simulink model "ModelCurrentState"  (R2024b)
settings: Solver=VariableStepAuto  StartTime=0.0  StopTime=StopTime  MaxStep=0.001  RelTol=1e-3
model workspace: external: MAT-File 3DModelInputs.mat (data not in the file)
undefined symbols (not defined in the file): GripStrength, KillswitchFinalValue, KillswitchInitialValue, KillswitchStepTime, LeftLowerArmLength, PlaneTilt, RightLowerArmLength, UpperTorsoLength, X, Y, Z
libraries: nesl_utility x408, sm_lib x139, matrix_library x11, simulink x1
(part 5 of 14)

== system ModelCurrentState/Right Shoulder Joint ==
  note: RSGlobal
  Dot Product1 : DotProduct  OutDataTypeStr=Inherit: Inherit via internal rule
  Dot Product2 : DotProduct  OutDataTypeStr=Inherit: Inherit via internal rule
  RArmonRSFGlobal : Gain  Gain=-1
  RArmonRSTGlobal : Gain  Gain=-1
  RS Kinematically Driven : Subsystem  Commented=on
  RS Kinetically Driven : Subsystem
  RSAV : nesl_utility/PS-Simulink Converter  PhysicalDomain=network_engine_domain  SubClassName=ps_output  LeftPortType=input  RightPortType=output  PseudoPeriodic=off  Frequencies=[]  VectorFormat=1-D array  Unit=deg/s  AffineConversion=off
  RSAngularWorkonArm : Integrator
  RSLinearImpulseonArm : Integrator
  RSLinearWorkonArm : Integrator
  RSgx : nesl_utility/PS-Simulink Converter  PhysicalDomain=network_engine_domain  SubClassName=ps_output  LeftPortType=input  RightPortType=output  PseudoPeriodic=off  Frequencies=[]  VectorFormat=1-D array  Unit=inherit  AffineConversion=off
  RSgy : nesl_utility/PS-Simulink Converter  PhysicalDomain=network_engine_domain  SubClassName=ps_output  LeftPortType=input  RightPortType=output  PseudoPeriodic=off  Frequencies=[]  VectorFormat=1-D array  Unit=inherit  AffineConversion=off
  RSgz : nesl_utility/PS-Simulink Converter  PhysicalDomain=network_engine_domain  SubClassName=ps_output  LeftPortType=input  RightPortType=output  PseudoPeriodic=off  Frequencies=[]  VectorFormat=1-D array  Unit=inherit  AffineConversion=off
  RSonRArmFGlob : Product  Multiplication=Matrix(*)
  RSonRArmLocalForce : nesl_utility/PS-Simulink Converter  PhysicalDomain=network_engine_domain  SubClassName=ps_output  LeftPortType=input  RightPortType=output  PseudoPeriodic=off  Frequencies=[]  VectorFormat=1-D array  Unit=inherit  AffineConversion=off
  RSonRArmLocalTorque : nesl_utility/PS-Simulink Converter  PhysicalDomain=network_engine_domain  SubClassName=ps_output  LeftPortType=input  RightPortType=output  PseudoPeriodic=off  Frequencies=[]  VectorFormat=1-D array  Unit=inherit  AffineConversion=off
  RSonRArmTGlobal : Product  Multiplication=Matrix(*)
  RSvGlobal : nesl_utility/PS-Simulink Converter  PhysicalDomain=network_engine_domain  SubClassName=ps_output  LeftPortType=input  RightPortType=output  PseudoPeriodic=off  Frequencies=[]  VectorFormat=1-D array  Unit=inherit  AffineConversion=off
  RSx : nesl_utility/PS-Simulink Converter  PhysicalDomain=network_engine_domain  SubClassName=ps_output  LeftPortType=input  RightPortType=output  PseudoPeriodic=off  Frequencies=[]  VectorFormat=1-D array  Unit=inherit  AffineConversion=off
  RSy : nesl_utility/PS-Simulink Converter  PhysicalDomain=network_engine_domain  SubClassName=ps_output  LeftPortType=input  RightPortType=output  PseudoPeriodic=off  Frequencies=[]  VectorFormat=1-D array  Unit=inherit  AffineConversion=off
  RSz : nesl_utility/PS-Simulink Converter  PhysicalDomain=network_engine_domain  SubClassName=ps_output  LeftPortType=input  RightPortType=output  PseudoPeriodic=off  Frequencies=[]  VectorFormat=1-D array  Unit=inherit  AffineConversion=off
  RotationMatrix : nesl_utility/PS-Simulink Converter  PhysicalDomain=network_engine_domain  SubClassName=ps_output  LeftPortType=input  RightPortType=output  PseudoPeriodic=off  Frequencies=[]  VectorFormat=1-D array  Unit=inherit  AffineConversion=off
  Spherical Solid : sm_lib/Body Elements/Spherical Solid  SphereRadius=1.75  SphereRadiusUnits=in  ExportEntireGeometry=off  InertiaType=CalculateFromGeometry  BasedOnType=Density  Density=0  DensityUnits=kg/m^3  Mass=1  MassUnits=kg  CenterOfMass=[0 0 0]  CenterOfMassUnits=m  MomentsOfInertia=[1 1 1]  MomentsOfInertiaUnits=kg*m^2  ProductsOfInertia=[0 0 0]  ProductsOfInertiaUnits=kg*m^2  GraphicType=FromGeometry  MarkerShape=Sphere  MarkerSize=10  GraphicVisPropType=SimpleVisualProperties  GraphicDiffuseColor=[0.2 0.2 1.0]  GraphicOpacity=1  GraphicSpecularColor=[0.5 0.5 0.5 1.0]  GraphicAmbientColor=[0.15 0.15 0.15 1.0]  GraphicEmissiveColor=[0.0 0.0 0.0 1.0]  GraphicShininess=75  DoExposeReferenceFrame=on  SerializedFrames=<Frames/>
  Transform Sensor : sm_lib/Frames and Transforms/Transform Sensor  MeasurementFrame=World  RotationSequence=XYX  SenseAngle=off  SenseAxis=off  SenseQ=off  SenseR=on  SenseRotationSequence=off  SenseOmegaX=off  SenseOmegaY=off  SenseOmegaZ=off  SenseOmega=off  SenseQDot=off  SenseRDot=off  SenseRotationSequenceDot=off  SenseAlphaX=off  SenseAlphaY=off  SenseAlphaZ=off  SenseAlpha=off  SenseQDDot=off  SenseRDDot=off  SenseX=on  SenseY=on  SenseZ=on  SenseXYZ=off  SenseRad=off  SenseAzim=off  SenseDist=off  SenseInc=off  SenseXDot=off  SenseYDot=off  SenseZDot=off  SenseXYZDot=off  SenseRadDot=off  SenseAzimDot=off  SenseDistDot=off  SenseIncDot=off  SenseXDDot=off  SenseYDDot=off  SenseZDDot=off  SenseXYZDDot=off  SenseRadDDot=off  SenseAzimDDot=off  SenseDistDDot=off  SenseIncDDot=off
  Transform Sensor1 : sm_lib/Frames and Transforms/Transform Sensor  MeasurementFrame=World  RotationSequence=XYX  SenseAngle=off  SenseAxis=off  SenseQ=off  SenseR=off  SenseRotationSequence=off  SenseOmegaX=off  SenseOmegaY=off  SenseOmegaZ=off  SenseOmega=on  SenseQDot=off  SenseRDot=off  SenseRotationSequenceDot=off  SenseAlphaX=off  SenseAlphaY=off  SenseAlphaZ=off  SenseAlpha=off  SenseQDDot=off  SenseRDDot=off  SenseX=on  SenseY=on  SenseZ=on  SenseXYZ=off  SenseRad=off  SenseAzim=off  SenseDist=off  SenseInc=off  SenseXDot=off  SenseYDot=off  SenseZDot=off  SenseXYZDot=on  SenseRadDot=off  SenseAzimDot=off  SenseDistDot=off  SenseIncDot=off  SenseXDDot=off  SenseYDDot=off  SenseZDDot=off  SenseXYZDDot=off  SenseRadDDot=off  SenseAzimDDot=off  SenseDistDDot=off  SenseIncDDot=off
  Vector Concatenate : Concatenate  NumInputs=3
  World Frame : sm_lib/Frames and Transforms/World Frame
  Right Shoulder : PMIOPort  Side=Left
  Top of Right Arm : PMIOPort  Port=2  Side=Right
  tag scope: RSGlobalPosition=global, RSonRArmFGlobalOut=global, RSonRArmTGlobalOut=global
  wires:
  RotationMatrix/1 -> RSonRArmFGlob/1, RSonRArmTGlobal/1
  RSonRArmLocalForce/1 -> RSonRArmFGlob/2
  RSonRArmLocalTorque/1 -> RSonRArmTGlobal/2
  RSonRArmTGlobal/1 -> Dot Product2/1, RArmonRSTGlobal/1, [RSonRArmTGlobalOut]  "RSonRArmTGlobal"
  RSgx/1 -> Vector Concatenate/1
  RSgy/1 -> Vector Concatenate/2
  Vector Concatenate/1 -> [RSGlobalPosition]  "RSGlobalPosition"
  RSgz/1 -> Vector Concatenate/3
  Dot Product1/1 -> RSLinearWorkonArm/1  "RSonArmLinearPower"
  Dot Product2/1 -> RSAngularWorkonArm/1  "RSonArmAngularPower"
  RSonRArmFGlob/1 -> RSLinearImpulseonArm/1, Dot Product1/1, [RSonRArmFGlobalOut], RArmonRSFGlobal/1  "RSonRArmFGlobal"
  RSvGlobal/1 -> Dot Product1/2  "RSVGlobal"
  RSAV/1 -> Dot Product2/2  "RSAVGlobal"
  connections:
  Spherical Solid/RConn1 -- RS Kinetically Driven/LConn1 -- Top of Right Arm/RConn1 -- RS Kinematically Driven/LConn1 -- Transform Sensor1/RConn1 -- Transform Sensor/RConn1
  RSgx/LConn1 -- Transform Sensor/RConn3
  RotationMatrix/LConn1 -- Transform Sensor/RConn2
  RSgz/LConn1 -- Transform Sensor/RConn5
  RSgy/LConn1 -- Transform Sensor/RConn4
  World Frame/RConn1 -- Transform Sensor1/LConn1 -- Transform Sensor/LConn1
  Transform Sensor1/RConn6 -- RSvGlobal/LConn1
  RSAV/LConn1 -- Transform Sensor1/RConn2
  Transform Sensor1/RConn5 -- RSz/LConn1
  Transform Sensor1/RConn4 -- RSy/LConn1
  Transform Sensor1/RConn3 -- RSx/LConn1
  RS Kinematically Driven/RConn1 -- Right Shoulder/RConn1 -- RS Kinetically Driven/RConn1
  RSonRArmLocalForce/LConn1 -- RS Kinetically Driven/RConn2
  RSonRArmLocalTorque/LConn1 -- RS Kinetically Driven/RConn3

== system ModelCurrentState/Right Upper Arm ==
  Cylindrical Solid3 : sm_lib/Body Elements/Cylindrical Solid  CylinderRadius=1.75  CylinderRadiusUnits=in  CylinderLength=12  CylinderLengthUnits=in  ExportEntireGeometry=off  InertiaType=CalculateFromGeometry  BasedOnType=Mass  Density=1000  DensityUnits=kg/m^3  Mass=5  MassUnits=lbm  CenterOfMass=[0 0 0]  CenterOfMassUnits=m  MomentsOfInertia=[1 1 1]  MomentsOfInertiaUnits=kg*m^2  ProductsOfInertia=[0 0 0]  ProductsOfInertiaUnits=kg*m^2  GraphicType=FromGeometry  MarkerShape=Sphere  MarkerSize=10  GraphicVisPropType=SimpleVisualProperties  GraphicDiffuseColor=[0.2 0.2 1.0]  GraphicOpacity=1.0  GraphicSpecularColor=[0.5 0.5 0.5 1.0]  GraphicAmbientColor=[0.15 0.15 0.15 1.0]  GraphicEmissiveColor=[0.0 0.0 0.0 1.0]  GraphicShininess=75  DoExposeReferenceFrame=off  SerializedFrames=<Frames><Frame><Id>Frame1</Id><Value><Name>Top of Right Arm</Name><Origin><Source>GeometricFeature</Source><FeatureName>top curve</FeatureName></Origin><PrimaryAxis><DefinedDirection>-X</DefinedDirection><Source>ReferenceFrame</Source><SourceDirection>+Z</SourceDirection><FeatureName></FeatureName></PrimaryAxis><SecondaryAxis><DefinedDirection>+Y</DefinedDirection><Source>ReferenceFrame</Source><SourceDirection>+X</SourceDirection><FeatureName></FeatureName></SecondaryAxis></Value></Frame><Frame><Id>Frame2</Id><Value><Name>Bottom of Right Arm</Name><Origin><Source>GeometricFeature</Source><FeatureName>bottom curve</FeatureName></Origin><PrimaryAxis><DefinedDirection>-X</DefinedDirection><Source>ReferenceFrame</Source><SourceDirection>+Z</SourceDirection><FeatureName></FeatureName></PrimaryAxis><SecondaryAxis><DefinedDirection>+Z</DefinedDirection><Source>ReferenceFrame</Source><SourceDirection>-X</SourceDirection><FeatureName></FeatureName></SecondaryAxis></Value></Frame></Frames>
  Right Upper Arm MOF : Subsystem  Commented=on
  RightUpper  Arm : PMIOPort  Side=Left
  Right Elbow : PMIOPort  Port=2  Side=Right
  connections:
  Right Upper Arm MOF/LConn1 -- RightUpper  Arm/RConn1 -- Cylindrical Solid3/LConn1
  Cylindrical Solid3/RConn1 -- Right Elbow/RConn1

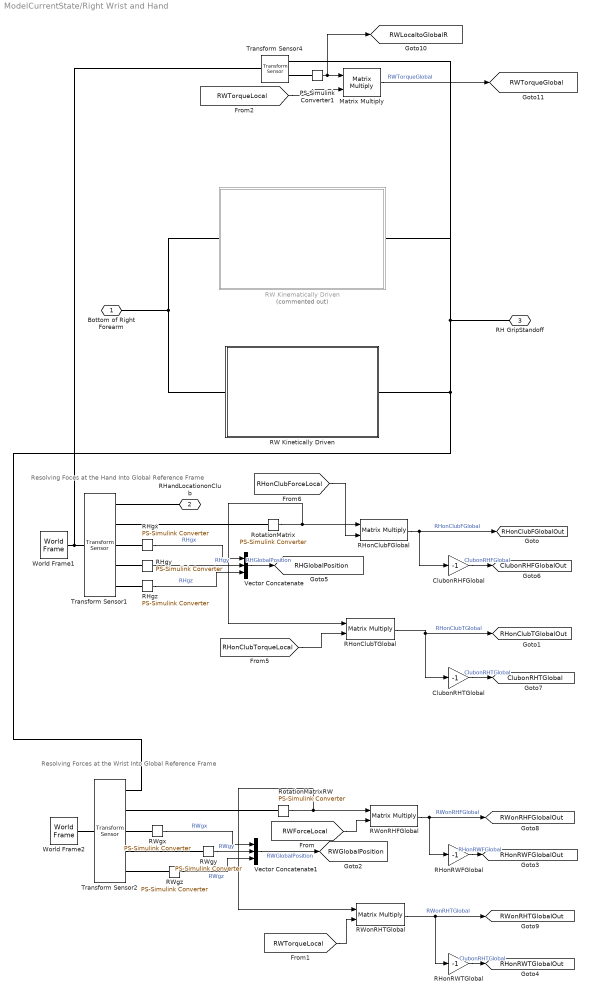
== system ModelCurrentState/Right Wrist and Hand ==
  note: Resolving Foces at the Hand Into Global Reference Frame
  note: Resolving Forces at the Wrist Into Global Reference Frame
  ClubonRHFGlobal : Gain  Gain=-1
  ClubonRHTGlobal : Gain  Gain=-1
  Matrix Multiply : Product  Multiplication=Matrix(*)
  PS-Simulink Converter1 : nesl_utility/PS-Simulink Converter  PhysicalDomain=network_engine_domain  SubClassName=ps_output  LeftPortType=input  RightPortType=output  PseudoPeriodic=off  Frequencies=[]  VectorFormat=1-D array  Unit=inherit  AffineConversion=off
  RHgx : nesl_utility/PS-Simulink Converter  PhysicalDomain=network_engine_domain  SubClassName=ps_output  LeftPortType=input  RightPortType=output  PseudoPeriodic=off  Frequencies=[]  VectorFormat=1-D array  Unit=inherit  AffineConversion=off
  RHgy : nesl_utility/PS-Simulink Converter  PhysicalDomain=network_engine_domain  SubClassName=ps_output  LeftPortType=input  RightPortType=output  PseudoPeriodic=off  Frequencies=[]  VectorFormat=1-D array  Unit=inherit  AffineConversion=off
  RHgz : nesl_utility/PS-Simulink Converter  PhysicalDomain=network_engine_domain  SubClassName=ps_output  LeftPortType=input  RightPortType=output  PseudoPeriodic=off  Frequencies=[]  VectorFormat=1-D array  Unit=inherit  AffineConversion=off
  RHonClubFGlobal : Product  Multiplication=Matrix(*)
  RHonClubTGlobal : Product  Multiplication=Matrix(*)
  RHonRWFGlobal : Gain  Gain=-1
  RHonRWTGlobal : Gain  Gain=-1
  RW Kinematically Driven : Subsystem  Commented=on
  RW Kinetically Driven : Subsystem
  RWgx : nesl_utility/PS-Simulink Converter  PhysicalDomain=network_engine_domain  SubClassName=ps_output  LeftPortType=input  RightPortType=output  PseudoPeriodic=off  Frequencies=[]  VectorFormat=1-D array  Unit=inherit  AffineConversion=off
  RWgy : nesl_utility/PS-Simulink Converter  PhysicalDomain=network_engine_domain  SubClassName=ps_output  LeftPortType=input  RightPortType=output  PseudoPeriodic=off  Frequencies=[]  VectorFormat=1-D array  Unit=inherit  AffineConversion=off
  RWgz : nesl_utility/PS-Simulink Converter  PhysicalDomain=network_engine_domain  SubClassName=ps_output  LeftPortType=input  RightPortType=output  PseudoPeriodic=off  Frequencies=[]  VectorFormat=1-D array  Unit=inherit  AffineConversion=off
  RWonRHFGlobal : Product  Multiplication=Matrix(*)
  RWonRHTGlobal : Product  Multiplication=Matrix(*)
  RotationMatrix : nesl_utility/PS-Simulink Converter  PhysicalDomain=network_engine_domain  SubClassName=ps_output  LeftPortType=input  RightPortType=output  PseudoPeriodic=off  Frequencies=[]  VectorFormat=1-D array  Unit=inherit  AffineConversion=off
  RotationMatrixRW : nesl_utility/PS-Simulink Converter  PhysicalDomain=network_engine_domain  SubClassName=ps_output  LeftPortType=input  RightPortType=output  PseudoPeriodic=off  Frequencies=[]  VectorFormat=1-D array  Unit=inherit  AffineConversion=off
  Transform Sensor1 : sm_lib/Frames and Transforms/Transform Sensor  MeasurementFrame=World  RotationSequence=XYX  SenseAngle=off  SenseAxis=off  SenseQ=off  SenseR=on  SenseRotationSequence=off  SenseOmegaX=off  SenseOmegaY=off  SenseOmegaZ=off  SenseOmega=off  SenseQDot=off  SenseRDot=off  SenseRotationSequenceDot=off  SenseAlphaX=off  SenseAlphaY=off  SenseAlphaZ=off  SenseAlpha=off  SenseQDDot=off  SenseRDDot=off  SenseX=on  SenseY=on  SenseZ=on  SenseXYZ=off  SenseRad=off  SenseAzim=off  SenseDist=off  SenseInc=off  SenseXDot=off  SenseYDot=off  SenseZDot=off  SenseXYZDot=off  SenseRadDot=off  SenseAzimDot=off  SenseDistDot=off  SenseIncDot=off  SenseXDDot=off  SenseYDDot=off  SenseZDDot=off  SenseXYZDDot=off  SenseRadDDot=off  SenseAzimDDot=off  SenseDistDDot=off  SenseIncDDot=off
  Transform Sensor2 : sm_lib/Frames and Transforms/Transform Sensor  MeasurementFrame=World  RotationSequence=XYX  SenseAngle=off  SenseAxis=off  SenseQ=off  SenseR=on  SenseRotationSequence=off  SenseOmegaX=off  SenseOmegaY=off  SenseOmegaZ=off  SenseOmega=off  SenseQDot=off  SenseRDot=off  SenseRotationSequenceDot=off  SenseAlphaX=off  SenseAlphaY=off  SenseAlphaZ=off  SenseAlpha=off  SenseQDDot=off  SenseRDDot=off  SenseX=on  SenseY=on  SenseZ=on  SenseXYZ=off  SenseRad=off  SenseAzim=off  SenseDist=off  SenseInc=off  SenseXDot=off  SenseYDot=off  SenseZDot=off  SenseXYZDot=off  SenseRadDot=off  SenseAzimDot=off  SenseDistDot=off  SenseIncDot=off  SenseXDDot=off  SenseYDDot=off  SenseZDDot=off  SenseXYZDDot=off  SenseRadDDot=off  SenseAzimDDot=off  SenseDistDDot=off  SenseIncDDot=off
  Transform Sensor4 : sm_lib/Frames and Transforms/Transform Sensor  MeasurementFrame=World  RotationSequence=XYX  SenseAngle=off  SenseAxis=off  SenseQ=off  SenseR=on  SenseRotationSequence=off  SenseOmegaX=off  SenseOmegaY=off  SenseOmegaZ=off  SenseOmega=off  SenseQDot=off  SenseRDot=off  SenseRotationSequenceDot=off  SenseAlphaX=off  SenseAlphaY=off  SenseAlphaZ=off  SenseAlpha=off  SenseQDDot=off  SenseRDDot=off  SenseX=off  SenseY=off  SenseZ=off  SenseXYZ=off  SenseRad=off  SenseAzim=off  SenseDist=off  SenseInc=off  SenseXDot=off  SenseYDot=off  SenseZDot=off  SenseXYZDot=off  SenseRadDot=off  SenseAzimDot=off  SenseDistDot=off  SenseIncDot=off  SenseXDDot=off  SenseYDDot=off  SenseZDDot=off  SenseXYZDDot=off  SenseRadDDot=off  SenseAzimDDot=off  SenseDistDDot=off  SenseIncDDot=off
  Vector Concatenate : Concatenate  NumInputs=3
  Vector Concatenate1 : Concatenate  NumInputs=3
  World Frame1 : sm_lib/Frames and Transforms/World Frame
  World Frame2 : sm_lib/Frames and Transforms/World Frame
  Bottom of Right Forearm : PMIOPort  Side=Left
  RHandLocationonClub : PMIOPort  Port=2  Side=Right
  RH GripStandoff : PMIOPort  Port=3  Side=Right
  tag scope: ClubonRHFGlobalOut=global, ClubonRHTGlobal=global, RHGlobalPosition=global, RHonClubFGlobalOut=global, RHonClubTGlobalOut=global, RHonRWFGlobalOut=global, RHonRWTGlobalOut=global, RWGlobalPosition=global, RWLocaltoGlobalR=global, RWTorqueGlobal=global, RWonRHFGlobalOut=global, RWonRHTGlobalOut=global
  wires:
  [RHonClubForceLocal] -> RHonClubFGlobal/2
  RotationMatrix/1 -> RHonClubTGlobal/1, RHonClubFGlobal/1
  ClubonRHFGlobal/1 -> [ClubonRHFGlobalOut]  "ClubonRHFGlobal"
  RHonClubFGlobal/1 -> ClubonRHFGlobal/1, [RHonClubFGlobalOut]  "RHonClubFGlobal"
  RHonClubTGlobal/1 -> ClubonRHTGlobal/1, [RHonClubTGlobalOut]  "RHonClubTGlobal"
  ClubonRHTGlobal/1 -> [ClubonRHTGlobal]  "ClubonRHTGlobal"
  RHgx/1 -> Vector Concatenate/1  "RHgx"
  RHgz/1 -> Vector Concatenate/3  "RHgz"
  RHgy/1 -> Vector Concatenate/2  "RHgy"
  [RHonClubTorqueLocal] -> RHonClubTGlobal/2
  RWgx/1 -> Vector Concatenate1/1  "RWgx"
  RHonRWTGlobal/1 -> [RHonRWTGlobalOut]  "ClubonRHTGlobal"
  RWonRHTGlobal/1 -> [RWonRHTGlobalOut], RHonRWTGlobal/1  "RWonRHTGlobal"
  RHonRWFGlobal/1 -> [RHonRWFGlobalOut]  "RHonRWFGlobal"
  RotationMatrixRW/1 -> RWonRHTGlobal/1, RWonRHFGlobal/1
  Vector Concatenate1/1 -> [RWGlobalPosition]  "RWGlobalPosition"
  RWgz/1 -> Vector Concatenate1/3  "RWgz"
  RWonRHFGlobal/1 -> RHonRWFGlobal/1, [RWonRHFGlobalOut]  "RWonRHFGlobal"
  RWgy/1 -> Vector Concatenate1/2  "RWgy"
  Vector Concatenate/1 -> [RHGlobalPosition]  "RHGlobalPosition"
  [RWForceLocal] -> RWonRHFGlobal/2
  [RWTorqueLocal] -> RWonRHTGlobal/2
  PS-Simulink Converter1/1 -> [RWLocaltoGlobalR], Matrix Multiply/1
  Matrix Multiply/1 -> [RWTorqueGlobal]  "RWTorqueGlobal"
  [RWTorqueLocal] -> Matrix Multiply/2
  connections:
  RotationMatrix/LConn1 -- Transform Sensor1/RConn2
  World Frame1/RConn1 -- Transform Sensor4/LConn1 -- Transform Sensor1/LConn1
  Transform Sensor1/RConn4 -- RHgy/LConn1
  Transform Sensor1/RConn5 -- RHgz/LConn1
  Transform Sensor1/RConn3 -- RHgx/LConn1
  RHandLocationonClub/RConn1 -- Transform Sensor1/RConn1
  Transform Sensor2/RConn5 -- RWgz/LConn1
  RotationMatrixRW/LConn1 -- Transform Sensor2/RConn2
  World Frame2/RConn1 -- Transform Sensor2/LConn1
  Transform Sensor2/RConn4 -- RWgy/LConn1
  Transform Sensor2/RConn3 -- RWgx/LConn1
  Transform Sensor2/RConn1 -- Transform Sensor4/RConn1 -- RW Kinematically Driven/RConn1 -- RH GripStandoff/RConn1 -- RW Kinetically Driven/RConn1
  RW Kinetically Driven/LConn1 -- RW Kinematically Driven/LConn1 -- Bottom of Right Forearm/RConn1
  Transform Sensor4/RConn2 -- PS-Simulink Converter1/LConn1

== system ModelCurrentState/Spine Input Function ==
  Spine Bending Torques : MATLAB Function  TreatAsAtomicUnit=on  SystemSampleTime=0
  tag scope: FcnOutSpineAccelerationX=global, FcnOutSpineAccelerationY=global, FcnOutSpinePositionX=global, FcnOutSpinePositionY=global, FcnOutSpineTorqueX=global, FcnOutSpineTorqueY=global, FcnOutSpineVelocityX=global, FcnOutSpineVelocityY=global
  wires:
  Spine Bending Torques/2(JointTorqueSpineY) -> [FcnOutSpineTorqueY]  "SpineTorqueYInput"
  [Time] -> Spine Bending Torques/1(Time)
  Spine Bending Torques/1(JointTorqueSpineX) -> [FcnOutSpineTorqueX]  "SpineTorqueXInput"
  [Killswitch] -> Spine Bending Torques/2(Killswitch)
  [SpineVelocityY] -> Spine Bending Torques/6(SpineVelocityY)
  [SpineVelocityX] -> Spine Bending Torques/5(SpineVelocityX)
  [SpinePositionY] -> Spine Bending Torques/4(SpinePositionY)
  [SpinePositionX] -> Spine Bending Torques/3(SpinePositionX)
  Spine Bending Torques/3(SpinePositionInputX) -> [FcnOutSpinePositionX]
  Spine Bending Torques/4(SpinePositionInputY) -> [FcnOutSpinePositionY]
  Spine Bending Torques/5(SpineVelocityInputX) -> [FcnOutSpineVelocityX]
  Spine Bending Torques/6(SpineVelocityInputY) -> [FcnOutSpineVelocityY]
  Spine Bending Torques/7(SpineAccelerationInputX) -> [FcnOutSpineAccelerationX]
  Spine Bending Torques/8(SpineAccelerationInputY) -> [FcnOutSpineAccelerationY]

== system ModelCurrentState/Torso Input Function ==
  Torso Input Torque : MATLAB Function  TreatAsAtomicUnit=on  SystemSampleTime=0
  tag scope: FcnOutTorsoAcceleration=global, FcnOutTorsoPosition=global, FcnOutTorsoTorque=global, FcnOutTorsoVelocity=global
  wires:
  [TorsoPosition] -> Torso Input Torque/3(TorsoPosition)  "TorsoPositionIn"
  Torso Input Torque/4(TorsoAccelerationInput) -> [FcnOutTorsoAcceleration]  "FcnOutTorsoAcceleration"
  [TorsoVelocity] -> Torso Input Torque/4(TorsoVelocity)  "TorsoVelocityIn"
  Torso Input Torque/1(JointTorqueTorso) -> [FcnOutTorsoTorque]  "TorsoTorqueInput"
  [Killswitch] -> Torso Input Torque/2(Killswitch)
  Torso Input Torque/2(TorsoPositionInput) -> [FcnOutTorsoPosition]  "FcnOutTorsoPosition"
  Torso Input Torque/3(TorsoVelocityInput) -> [FcnOutTorsoVelocity]  "FcnOutTorsoVelocity"
  [Time] -> Torso Input Torque/1(Time)

== system ModelCurrentState/Translation Input Function ==
  ConvertGlobalXtoHipBaseLocal : Product  Multiplication=Matrix(*)
  Demux : Demux  Outputs=3
  GlobalBaseTranslationalForce : MATLAB Function  TreatAsAtomicUnit=on  SystemSampleTime=0
  Mux : Mux  Inputs=3
  tag scope: FcnOutTranslationAccelerationX=global, FcnOutTranslationAccelerationY=global, FcnOutTranslationAccelerationZ=global, FcnOutTranslationForceX=global, FcnOutTranslationForceY=global, FcnOutTranslationForceZ=global, FcnOutTranslationPositionX=global, FcnOutTranslationPositionY=global, FcnOutTranslationPositionZ=global, FcnOutTranslationVelocityX=global, FcnOutTranslationVelocityY=global, FcnOutTranslationVelocityZ=global
  wires:
  Mux/1 -> ConvertGlobalXtoHipBaseLocal/2
  [Killswitch] -> GlobalBaseTranslationalForce/2(Killswitch)
  ConvertGlobalXtoHipBaseLocal/1 -> Demux/1  "BaseonHipForceHipBase"
  GlobalBaseTranslationalForce/8(TranslationVelocityInputY) -> [FcnOutTranslationVelocityY]
  GlobalBaseTranslationalForce/3(TranslationForceZ) -> Mux/3  "TranslationForceZInput"
  GlobalBaseTranslationalForce/1(TranslationForceX) -> Mux/1  "TranslationForceXInput"
  GlobalBaseTranslationalForce/11(TranslationAccelerationInputY) -> [FcnOutTranslationAccelerationY]
  Demux/3 -> [FcnOutTranslationForceZ]  "BaseonHipForceHipBaseZ"
  GlobalBaseTranslationalForce/2(TranslationForceY) -> Mux/2  "TranslationForceYInput"
  GlobalBaseTranslationalForce/5(TranslationPositionInputY) -> [FcnOutTranslationPositionY]
  GlobalBaseTranslationalForce/4(TranslationPositionInputX) -> [FcnOutTranslationPositionX]
  GlobalBaseTranslationalForce/10(TranslationAccelerationInputX) -> [FcnOutTranslationAccelerationX]
  Demux/2 -> [FcnOutTranslationForceY]  "BaseonHipForceHipBaseY"
  GlobalBaseTranslationalForce/12(TranslationAccelerationInputZ) -> [FcnOutTranslationAccelerationZ]
  [RotationMatrixGlobaltoHipJointBase] -> ConvertGlobalXtoHipBaseLocal/1
  GlobalBaseTranslationalForce/9(TranslationVelocityInputZ) -> [FcnOutTranslationVelocityZ]
  [Time] -> GlobalBaseTranslationalForce/1(Time)
  Demux/1 -> [FcnOutTranslationForceX]  "BaseonHipForceHipBaseX"
  GlobalBaseTranslationalForce/7(TranslationVelocityInputX) -> [FcnOutTranslationVelocityX]
  GlobalBaseTranslationalForce/6(TranslationPositionInputZ) -> [FcnOutTranslationPositionZ]
  [HipGlobalPositionX] -> GlobalBaseTranslationalForce/3(TranslationPositionX)
  [HipGlobalPositionY] -> GlobalBaseTranslationalForce/4(TranslationPositionY)
  [HipGlobalPositionZ] -> GlobalBaseTranslationalForce/5(TranslationPositionZ)
  [HipGlobalVelocityX] -> GlobalBaseTranslationalForce/6(TranslationVelocityX)
  [HipGlobalVelocityY] -> GlobalBaseTranslationalForce/7(TranslationVelocityY)
  [HipGlobalVelocityZ] -> GlobalBaseTranslationalForce/8(TranslationVelocityZ)

== system ModelCurrentState/Club/Flexible Beam Model ==
  Flexible Cylindrical Beam : sm_lib/Body Elements/Flexible Bodies/Beams/Flexible Cylindrical Beam  SectionType=Hollow  Radius=0.010  RadiusUnits=m  Thickness=0.0015  ThicknessUnits=m  Length=ShaftLength  LengthUnits=m  StiffnessAndInertiaType=CalculateFromGeometry  Density=500  DensityUnits=kg/m^3  ModuliType=YoungsPoissons  YoungsModulus=ShaftStiffness  YoungsModulusUnits=GPa  PoissonsRatio=0.33  ShearModulus=26  ShearModulusUnits=GPa  GeometricCentroid=[0 0]  GeometricCentroidUnits=m  BendingCentroid=[0 0]  BendingCentroidUnits=m  ShearCenter=[0 0]  ShearCenterUnits=m  AxialRigidity=1  AxialRigidityUnits=Pa*m^2  FlexuralRigidity=[1 1]  FlexuralRigidityUnits=Pa*m^4  CrossFlexuralRigidity=0  CrossFlexuralRigidityUnits=Pa*m^4  TorsionalRigidity=1  TorsionalRigidityUnits=Pa*m^4  CenterOfMass=[0 0]  CenterOfMassUnits=m  MassPerUnitLength=1  MassPerUnitLengthUnits=kg/m  MassMomentOfInertiaDensity=[1 1]  MassMomentOfInertiaDensityUnits=kg*m  MassProductOfInertiaDensity=0  MassProductOfInertiaDensityUnits=kg*m  DampingType=Proportional  ProportionalDampingAlpha=0  ProportionalDampingAlphaUnits=1/s  ProportionalDampingBeta=ShaftDampening  ProportionalDampingBetaUnits=s  UniformModalDampingRatio=0.01  NumElements=1  ReductionType=None  NumRetainedModes=1  GraphicType=FromGeometry  GraphicVisPropType=SimpleVisualProperties  GraphicDiffuseColor=[0.5 0.5 0.5]  GraphicOpacity=1.0  GraphicSpecularColor=[0.5 0.5 0.5 1.0]  GraphicAmbientColor=[0.15 0.15 0.15 1.0]  GraphicEmissiveColor=[0.0 0.0 0.0 1.0]  GraphicShininess=75  DoExposeZminFrame=on  DoExposeZmaxFrame=on  SerializedFrames=<Frames/>
  Rigid Transform : sm_lib/Frames and Transforms/Rigid Transform  RotationMethod=RotationSequence  FollAlignAxisA=+X  BaseAlignAxisA=+Y  FollAlignAxisB=+Y  BaseAlignAxisB=+Z  RotationStandardAxis=+Z  RotationAngle=0.0  RotationAngleUnits=deg  RotationArbitraryAxis=[0 0 1]  RotationSequenceAxes=FollowerAxes  RotationSequence=XYX  RotationSequenceAngles=[0 90 0]  RotationSequenceAnglesUnits=deg  RotationMatrix=[1 0 0; 0 1 0; 0 0 1]  Quaternion=[1 0 0 0]  TranslationMethod=None  TranslationCartesianOffset=[0 0 0]  TranslationCartesianOffsetUnits=m  TranslationStandardAxis=+Z  TranslationStandardOffset=0  TranslationStandardOffsetUnits=m  TranslationROffset=0  TranslationROffsetUnits=m  TranslationThetaOffset=0  TranslationThetaOffsetUnits=deg  TranslationZOffset=0  TranslationZOffsetUnits=m
  RH Grip : PMIOPort  Side=Left
  Clubhead : PMIOPort  Port=2  Side=Right
  connections:
  Rigid Transform/RConn1 -- Flexible Cylindrical Beam/LConn1
  RH Grip/RConn1 -- Rigid Transform/LConn1
  Flexible Cylindrical Beam/RConn1 -- Clubhead/RConn1

== system ModelCurrentState/Club/Rigid Shaft ==
  Rigid Shaft : sm_lib/Body Elements/Cylindrical Solid  CylinderRadius=0.01  CylinderRadiusUnits=m  CylinderLength=1  CylinderLengthUnits=m  ExportEntireGeometry=off  InertiaType=CalculateFromGeometry  BasedOnType=Mass  Density=500  DensityUnits=kg/m^3  Mass=0.0802566  MassUnits=kg  CenterOfMass=[0 0 0]  CenterOfMassUnits=m  MomentsOfInertia=[1 1 1]  MomentsOfInertiaUnits=kg*m^2  ProductsOfInertia=[0 0 0]  ProductsOfInertiaUnits=kg*m^2  GraphicType=FromGeometry  MarkerShape=Sphere  MarkerSize=10  GraphicVisPropType=SimpleVisualProperties  GraphicDiffuseColor=[0.5 0.5 0.5]  GraphicOpacity=1.0  GraphicSpecularColor=[0.5 0.5 0.5 1.0]  GraphicAmbientColor=[0.15 0.15 0.15 1.0]  GraphicEmissiveColor=[0.0 0.0 0.0 1.0]  GraphicShininess=75  DoExposeReferenceFrame=off  SerializedFrames=<Frames><Frame><Id>Frame1</Id><Value><Name>RHGripTOS</Name><Origin><Source>GeometricFeature</Source><FeatureName>top curve</FeatureName></Origin><PrimaryAxis><DefinedDirection>-X</DefinedDirection><Source>ReferenceFrame</Source><SourceDirection>+Z</SourceDirection><FeatureName></FeatureName></PrimaryAxis><SecondaryAxis><DefinedDirection>+Y</DefinedDirection><Source>ReferenceFrame</Source><SourceDirection>+X</SourceDirection><FeatureName></FeatureName></SecondaryAxis></Value></Frame><Frame><Id>Frame2</Id><Value><Name>ShaftS1</Name><Origin><Source>GeometricFeature</Source><FeatureName>bottom curve</FeatureName></Origin><PrimaryAxis><DefinedDirection>-X</DefinedDirection><Source>ReferenceFrame</Source><SourceDirection>+Z</SourceDirection><FeatureName></FeatureName></PrimaryAxis><SecondaryAxis><DefinedDirection>+Y</DefinedDirection><Source>ReferenceFrame</Source><SourceDirection>+X</SourceDirection><FeatureName></FeatureName></SecondaryAxis></Value></Frame></Frames>
  RH : PMIOPort  Side=Right
  Clubhead : PMIOPort  Port=2  Side=Right
  connections:
  RH/RConn1 -- Rigid Shaft/LConn1
  Clubhead/RConn1 -- Rigid Shaft/RConn1

== system ModelCurrentState/Club/Zero Mass Reference Shaft ==
  CHSCalculation : Subsystem  Commented=on
  CHvx : nesl_utility/PS-Simulink Converter  Commented=on  PhysicalDomain=network_engine_domain  SubClassName=ps_output  LeftPortType=input  RightPortType=output  PseudoPeriodic=off  Frequencies=[]  VectorFormat=1-D array  Unit=inherit  AffineConversion=off
  CHvy : nesl_utility/PS-Simulink Converter  Commented=on  PhysicalDomain=network_engine_domain  SubClassName=ps_output  LeftPortType=input  RightPortType=output  PseudoPeriodic=off  Frequencies=[]  VectorFormat=1-D array  Unit=inherit  AffineConversion=off
  CHvz : nesl_utility/PS-Simulink Converter  Commented=on  PhysicalDomain=network_engine_domain  SubClassName=ps_output  LeftPortType=input  RightPortType=output  PseudoPeriodic=off  Frequencies=[]  VectorFormat=1-D array  Unit=inherit  AffineConversion=off
  CHx : nesl_utility/PS-Simulink Converter  Commented=on  PhysicalDomain=network_engine_domain  SubClassName=ps_output  LeftPortType=input  RightPortType=output  PseudoPeriodic=off  Frequencies=[]  VectorFormat=1-D array  Unit=inherit  AffineConversion=off
  CHy : nesl_utility/PS-Simulink Converter  Commented=on  PhysicalDomain=network_engine_domain  SubClassName=ps_output  LeftPortType=input  RightPortType=output  PseudoPeriodic=off  Frequencies=[]  VectorFormat=1-D array  Unit=inherit  AffineConversion=off
  CHz : nesl_utility/PS-Simulink Converter  Commented=on  PhysicalDomain=network_engine_domain  SubClassName=ps_output  LeftPortType=input  RightPortType=output  PseudoPeriodic=off  Frequencies=[]  VectorFormat=1-D array  Unit=inherit  AffineConversion=off
  ClubheadPathUnitVector : Mux  Commented=on  Inputs=3
  ShaftPhysicalConfig : Subsystem
  Transform Sensor : sm_lib/Frames and Transforms/Transform Sensor  Commented=on  MeasurementFrame=World  RotationSequence=XYX  SenseAngle=off  SenseAxis=off  SenseQ=off  SenseR=off  SenseRotationSequence=off  SenseOmegaX=off  SenseOmegaY=off  SenseOmegaZ=off  SenseOmega=off  SenseQDot=off  SenseRDot=off  SenseRotationSequenceDot=off  SenseAlphaX=off  SenseAlphaY=off  SenseAlphaZ=off  SenseAlpha=off  SenseQDDot=off  SenseRDDot=off  SenseX=on  SenseY=on  SenseZ=on  SenseXYZ=off  SenseRad=off  SenseAzim=off  SenseDist=off  SenseInc=off  SenseXDot=on  SenseYDot=on  SenseZDot=on  SenseXYZDot=off  SenseRadDot=off  SenseAzimDot=off  SenseDistDot=off  SenseIncDot=off  SenseXDDot=off  SenseYDDot=off  SenseZDDot=off  SenseXYZDDot=off  SenseRadDDot=off  SenseAzimDDot=off  SenseDistDDot=off  SenseIncDDot=off
  UnitVectorX : Product  Commented=on  Inputs=*/
  UnitVectorY : Product  Commented=on  Inputs=*/
  UnitVectorZ : Product  Commented=on  Inputs=*/
  RH : PMIOPort  Side=Right
  ConnGlobal : PMIOPort  Port=2  Side=Right
  wires:
  CHvz/1 -> CHSCalculation/3(In1), UnitVectorZ/1
  CHvy/1 -> CHSCalculation/2(In3), UnitVectorY/1
  UnitVectorY/1 -> ClubheadPathUnitVector/2
  UnitVectorZ/1 -> ClubheadPathUnitVector/3
  CHSCalculation/1(Out1) -> UnitVectorY/2, UnitVectorZ/2, UnitVectorX/2  "GhostCHS"
  UnitVectorX/1 -> ClubheadPathUnitVector/1
  CHvx/1 -> CHSCalculation/1(In2), UnitVectorX/1
  connections:
  ShaftPhysicalConfig/RConn1 -- RH/RConn1
  ConnGlobal/RConn1 -- Transform Sensor/LConn1
  ShaftPhysicalConfig/RConn2 -- Transform Sensor/RConn1
  CHy/LConn1 -- Transform Sensor/RConn3
  CHvy/LConn1 -- Transform Sensor/RConn6
  CHx/LConn1 -- Transform Sensor/RConn2
  CHz/LConn1 -- Transform Sensor/RConn4
  CHvz/LConn1 -- Transform Sensor/RConn7
  CHvx/LConn1 -- Transform Sensor/RConn5

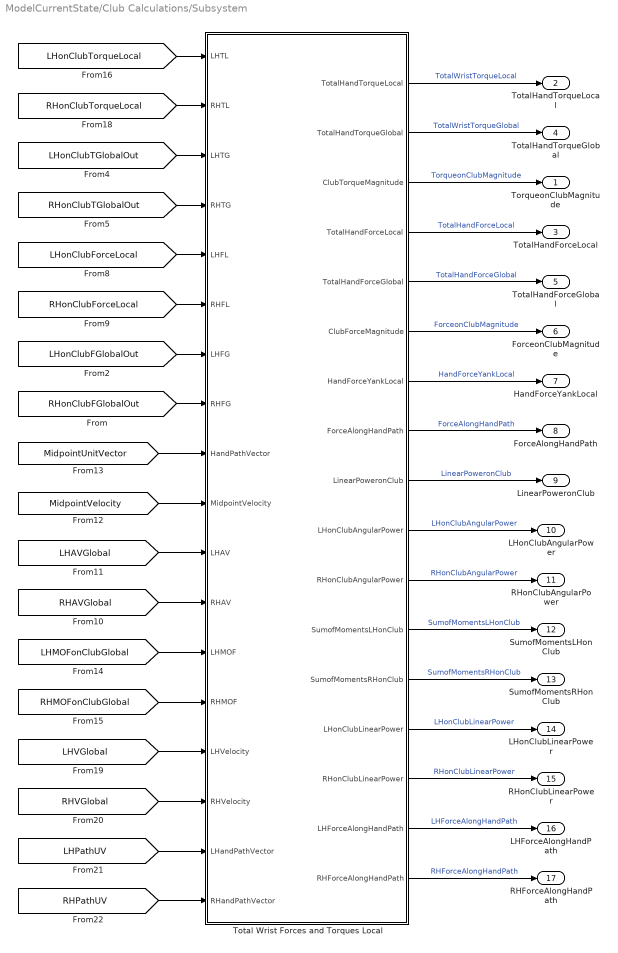
== system ModelCurrentState/Club Calculations/Subsystem ==
  Total Wrist Forces and Torques Local : MATLAB Function  TreatAsAtomicUnit=on  SystemSampleTime=0
  TorqueonClubMagnitude : Outport  PortDimensions=1
  TotalHandTorqueLocal : Outport  Port=2  PortDimensions=3
  TotalHandForceLocal : Outport  Port=3  PortDimensions=3
  TotalHandTorqueGlobal : Outport  Port=4  PortDimensions=3
  TotalHandForceGlobal : Outport  Port=5  PortDimensions=3
  ForceonClubMagnitude : Outport  Port=6  PortDimensions=1
  HandForceYankLocal : Outport  Port=7  PortDimensions=2
  ForceAlongHandPath : Outport  Port=8  PortDimensions=1
  LinearPoweronClub : Outport  Port=9  PortDimensions=1
  LHonClubAngularPower : Outport  Port=10  PortDimensions=1
  RHonClubAngularPower : Outport  Port=11  PortDimensions=1
  SumofMomentsLHonClub : Outport  Port=12  PortDimensions=3
  SumofMomentsRHonClub : Outport  Port=13  PortDimensions=3
  LHonClubLinearPower : Outport  Port=14  PortDimensions=1
  RHonClubLinearPower : Outport  Port=15
  LHForceAlongHandPath : Outport  Port=16  PortDimensions=1
  RHForceAlongHandPath : Outport  Port=17  PortDimensions=1
  wires:
  [LHonClubTGlobalOut] -> Total Wrist Forces and Torques Local/3(LHTG)
  [MidpointUnitVector] -> Total Wrist Forces and Torques Local/9(HandPathVector)
  [RHonClubForceLocal] -> Total Wrist Forces and Torques Local/6(RHFL)
  [RHonClubTorqueLocal] -> Total Wrist Forces and Torques Local/2(RHTL)
  [LHonClubFGlobalOut] -> Total Wrist Forces and Torques Local/7(LHFG)
  [LHonClubForceLocal] -> Total Wrist Forces and Torques Local/5(LHFL)
  [RHAVGlobal] -> Total Wrist Forces and Torques Local/12(RHAV)
  [LHPathUV] -> Total Wrist Forces and Torques Local/17(LHandPathVector)
  [RHonClubTGlobalOut] -> Total Wrist Forces and Torques Local/4(RHTG)
  [MidpointVelocity] -> Total Wrist Forces and Torques Local/10(MidpointVelocity)
  [LHVGlobal] -> Total Wrist Forces and Torques Local/15(LHVelocity)
  [RHVGlobal] -> Total Wrist Forces and Torques Local/16(RHVelocity)
  [RHonClubFGlobalOut] -> Total Wrist Forces and Torques Local/8(RHFG)
  Total Wrist Forces and Torques Local/15(RHonClubLinearPower) -> RHonClubLinearPower/1  "RHonClubLinearPower"
  Total Wrist Forces and Torques Local/4(TotalHandForceLocal) -> TotalHandForceLocal/1  "TotalHandForceLocal"
  [RHPathUV] -> Total Wrist Forces and Torques Local/18(RHandPathVector)
  [LHMOFonClubGlobal] -> Total Wrist Forces and Torques Local/13(LHMOF)
  [LHAVGlobal] -> Total Wrist Forces and Torques Local/11(LHAV)
  Total Wrist Forces and Torques Local/5(TotalHandForceGlobal) -> TotalHandForceGlobal/1  "TotalHandForceGlobal"
  [LHonClubTorqueLocal] -> Total Wrist Forces and Torques Local/1(LHTL)
  Total Wrist Forces and Torques Local/6(ClubForceMagnitude) -> ForceonClubMagnitude/1  "ForceonClubMagnitude"
  Total Wrist Forces and Torques Local/7(HandForceYankLocal) -> HandForceYankLocal/1  "HandForceYankLocal"
  [RHMOFonClubGlobal] -> Total Wrist Forces and Torques Local/14(RHMOF)
  Total Wrist Forces and Torques Local/13(SumofMomentsRHonClub) -> SumofMomentsRHonClub/1  "SumofMomentsRHonClub"
  Total Wrist Forces and Torques Local/16(LHForceAlongHandPath) -> LHForceAlongHandPath/1  "LHForceAlongHandPath"
  Total Wrist Forces and Torques Local/12(SumofMomentsLHonClub) -> SumofMomentsLHonClub/1  "SumofMomentsLHonClub"
  Total Wrist Forces and Torques Local/9(LinearPoweronClub) -> LinearPoweronClub/1  "LinearPoweronClub"
  Total Wrist Forces and Torques Local/8(ForceAlongHandPath) -> ForceAlongHandPath/1  "ForceAlongHandPath"
  Total Wrist Forces and Torques Local/14(LHonClubLinearPower) -> LHonClubLinearPower/1  "LHonClubLinearPower"
  Total Wrist Forces and Torques Local/11(RHonClubAngularPower) -> RHonClubAngularPower/1  "RHonClubAngularPower"
  Total Wrist Forces and Torques Local/3(ClubTorqueMagnitude) -> TorqueonClubMagnitude/1  "TorqueonClubMagnitude"
  Total Wrist Forces and Torques Local/10(LHonClubAngularPower) -> LHonClubAngularPower/1  "LHonClubAngularPower"
  Total Wrist Forces and Torques Local/2(TotalHandTorqueGlobal) -> TotalHandTorqueGlobal/1  "TotalWristTorqueGlobal"
  Total Wrist Forces and Torques Local/1(TotalHandTorqueLocal) -> TotalHandTorqueLocal/1  "TotalWristTorqueLocal"
  Total Wrist Forces and Torques Local/17(RHForceAlongHandPath) -> RHForceAlongHandPath/1  "RHForceAlongHandPath"

== system ModelCurrentState/Club Calculations/Work and Impulse Integrators ==
  LHLinearWorkonClub : Integrator
  LWAngularImpulseonClub : Integrator
  LWAngularWorkonClub : Integrator
  LeftHandLinearImpulse : Integrator
  LinearImpulseonClub : Integrator
  LinearWorkonClub : Integrator
  RHLinearWorkOnClub : Integrator
  RWAngularImpulseonClub : Integrator
  RWAngularWorkonClub : Integrator
  RightHandLinearImpulseonClub : Integrator
  wires:
  [TotalHandForceGlobal] -> LinearImpulseonClub/1
  [LHonClubLinearPower] -> LHLinearWorkonClub/1
  [LinearPoweronClub] -> LinearWorkonClub/1
  [RHonClubAngularPower] -> RWAngularWorkonClub/1
  [RHonClubFGlobalOut] -> RightHandLinearImpulseonClub/1
  [LHonClubFGlobalOut] -> LeftHandLinearImpulse/1
  [LHonClubAngularPower] -> LWAngularWorkonClub/1
  [SumofMomentsRHonClub] -> RWAngularImpulseonClub/1
  [SumofMomentsLHonClub] -> LWAngularImpulseonClub/1
  [RHonClubLinearPower] -> RHLinearWorkOnClub/1
